simulink model "RocketTrajectory_TestModel"  (R2014a)
settings: Solver=ode3  StartTime=0.0  StopTime=25  FixedStep=0.01  MinStep=0.01  RelTol=1e-3
undefined symbols (not defined in the file or in its folder): area_rocket_planform, distance_tip_to_COP, dry_motor_weight, dry_rocket_cog, dry_rocket_weight, ground_launch_altitude, ground_pressure_ambient, ground_temperature_ambient, launch_angle, mass_flow_rate, moment_inertia_rocket, wet_motor_mass, wet_motor_weight
libraries: rocket_vertical_flight_library x4, rocket_drag_library x3, rocket_isa_model_library x2, rocket_dynamic_data_library x2, rocket_angular_flight_library x2
settings Model: Creator=scorpii  LastModifiedBy=scorpii
settings SolverCC: InitialStep=0.01
settings DataIOCC: LimitDataPoints=off
settings OptimizationCC: SimCompilerOptimization=off
settings DebuggingCC: ArtificialAlgebraicLoopMsg=error  MergeDetectMultiDrivingBlocksExec=error  FrameProcessingCompatibilityMsg=error
settings RTWCC: RTWCompilerOptimization=off

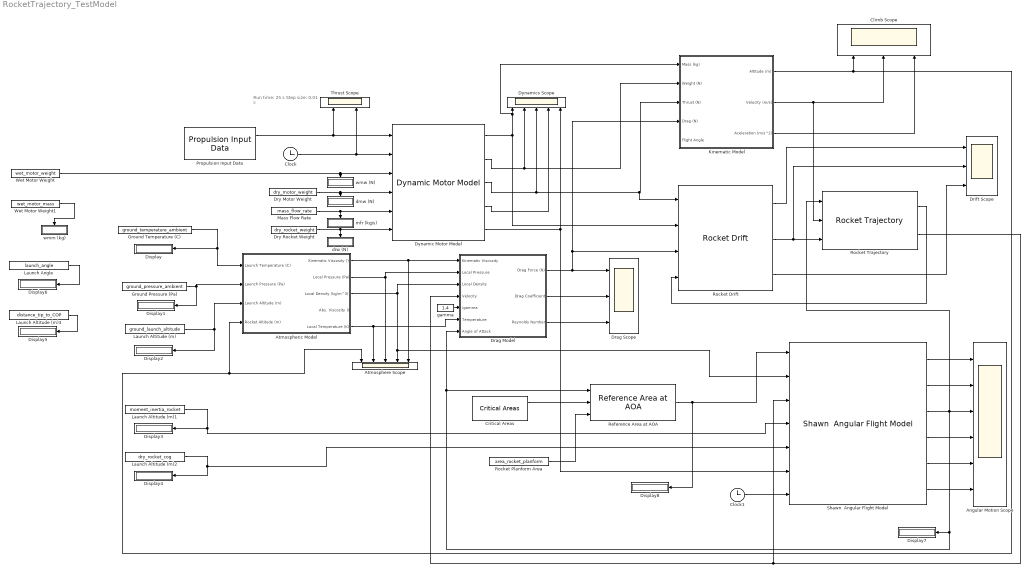
== system RocketTrajectory_TestModel ==
  note: Run time: 25 s
      | Step size: 0.01 s
  " Launch Angle" : Constant  Value=launch_angle
  Angular Motion Scope : Scope  NumInputPorts=6
      settings: TimeRange=10  YMin=-0.7~-0.125~-0.015~0.05~9~-5  YMax=0.9~0.125~0.015~0.275~24~5  SaveName=ScopeData5
  Atmosphere Scope : Scope  NumInputPorts=5
      settings: YMin=-1~28.5~96258.8~11.1784~-1.12485e-07  YMax=1~31.5~106391~12.355~-1.01773e-07  SaveName=ScopeData4
  Atmospheric Model : Subsystem
  Climb Scope : Scope  NumInputPorts=3
      settings: YMin=5.2~32.5~103.575  YMax=7~37.75~104.15
  Clock : Clock
  Clock1 : Clock
  Critical Areas : rocket_drag_library/Critical Areas
  Display{,1..8} (9 alike) : Display
  Drag Model : Subsystem
  Drag Scope : Scope  NumInputPorts=3
      settings: YMin=30~0.45~1.75e+07  YMax=240~0.725~5e+07  SaveName=ScopeData3
  Drift Scope : Scope  NumInputPorts=3
      settings: YMin=5.2~32.5~103.575  YMax=7~37.75~104.15  SaveName=ScopeData6
  Dry Motor Weight : Constant  Value=dry_motor_weight
  Dry Rocket Weight : Constant  Value=dry_rocket_weight
  Dynamic Motor Model : rocket_dynamic_data_library/Dynamic Motor Model
  Dynamics Scope : Scope  NumInputPorts=5
      settings: YMin=126.243~1238.44~774.486~-5~-5  YMax=139.531~1368.8~856.01~5~5
  Ground Pressure (Pa) : Constant  Value=ground_pressure_ambient
  Ground Temperature (C) : Constant  Value=ground_temperature_ambient
  Kinematic Model : Subsystem
  Launch Altitude (m) : Constant  Value=ground_launch_altitude
  Launch Altitude (m)1 : Constant  Value=moment_inertia_rocket
  Launch Altitude (m)2 : Constant  Value=dry_rocket_cog
  Launch Altitude (m)3 : Constant  Value=distance_tip_to_COP
  Mass Flow Rate : Constant  Value=mass_flow_rate
  Propulsion Input Data : rocket_dynamic_data_library/Propulsion Input Data
  Reference Area at AOA : rocket_angular_flight_library/Reference Area at AOA
  Rocket Drift : rocket_vertical_flight_library/Rocket Drift
  Rocket Planform Area : Constant  Value=area_rocket_planform
  Rocket Trajectory : rocket_vertical_flight_library/Rocket Trajectory
  Shawn  Angular Flight Model : rocket_angular_flight_library/Shawn  Angular Flight Model
  Thrust Scope : Scope  NumInputPorts=2
      settings: YMin=126.243~1238.44  YMax=139.531~1368.8  SaveName=ScopeData2
  "Wet Motor Weight " : Constant  Value=wet_motor_weight
  Wet Motor Weight1 : Constant  Value=wet_motor_mass
  dmw (N) : Display
  drw (N) : Display
  gamma : Constant  Value=1.4
  mfr (kg/s) : Display
  wmm (kg) : Display
  wmw (N) : Display
  wires:
  Drag Model/1(Drag Force (N)) -> Drag Scope/1, Rocket Drift/3, Kinematic Model/4(Drag (N))
  Clock/1 -> Dynamic Motor Model/2, Thrust Scope/2
  Kinematic Model/1(Altitude (m)) -> Climb Scope/1, Atmosphere Scope/1, Atmospheric Model/4(Rocket Altitude (m))
  Kinematic Model/2(Velocity (m/s)) -> Climb Scope/2, Rocket Trajectory/2
  Kinematic Model/3(Aceleration (m/s^2)) -> Climb Scope/3
  Atmospheric Model/3(Local Density (kg/m^3)) -> Shawn  Angular Flight Model/2, Atmosphere Scope/4, Drag Model/3(Local Density)
  Atmospheric Model/2(Local Pressure (Pa)) -> Atmosphere Scope/3, Drag Model/2(Local Pressure)
  Atmospheric Model/1(Kinematic Viscosity ()) -> Atmosphere Scope/5, Drag Model/1(Kinematic Viscosity)
  Atmospheric Model/5(Local Temperature (K)) -> Atmosphere Scope/2, Drag Model/6(Temperature)
  Dynamic Motor Model/2 -> Kinematic Model/2(Weight (N)), Dynamics Scope/2
  Dynamic Motor Model/1 -> Rocket Drift/2, Kinematic Model/1(Mass (kg)), Dynamics Scope/1
  Dynamic Motor Model/3 -> Rocket Drift/1, Kinematic Model/3(Thrust (N)), Dynamics Scope/3
  Propulsion Input Data/1 -> Dynamic Motor Model/1, Thrust Scope/1
  "Wet Motor Weight "/1 -> Dynamic Motor Model/3, wmw (N)/1
  Dry Motor Weight/1 -> Dynamic Motor Model/4, dmw (N)/1
  Mass Flow Rate/1 -> Dynamic Motor Model/5, mfr (kg/s)/1
  Drag Model/2(Drag Coefficient) -> Drag Scope/2
  Drag Model/3(Reynolds Number) -> Drag Scope/3
  gamma/1 -> Drag Model/5(\gamma)
  Ground Temperature (C)/1 -> Display/1, Atmospheric Model/1(Launch Temperature (C))
  Ground Pressure (Pa)/1 -> Display1/1, Atmospheric Model/2(Launch Pressure (Pa))
  Launch Altitude (m)/1 -> Atmospheric Model/3(Launch Altitude (m)), Display2/1
  Dynamic Motor Model/4 -> Dynamics Scope/4
  Dry Rocket Weight/1 -> Dynamic Motor Model/6, drw (N)/1
  Launch Altitude (m)1/1 -> Display3/1, Shawn  Angular Flight Model/4
  Shawn  Angular Flight Model/3 -> Rocket Trajectory/1, Display7/1, Drag Model/7(Angle of Attack), Reference Area at AOA/1, Angular Motion Scope/3
  Launch Altitude (m)2/1 -> Shawn  Angular Flight Model/5, Display4/1
  Launch Altitude (m)3/1 -> Display5/1
  Rocket Planform Area/1 -> Reference Area at AOA/3
  Critical Areas/1 -> Reference Area at AOA/2
  " Launch Angle"/1 -> Display6/1
  Shawn  Angular Flight Model/2 -> Angular Motion Scope/2
  Shawn  Angular Flight Model/1 -> Angular Motion Scope/1
  Wet Motor Weight1/1 -> wmm (kg)/1
  Reference Area at AOA/1 -> Display8/1, Shawn  Angular Flight Model/1
  Dynamic Motor Model/5 -> Shawn  Angular Flight Model/6, Dynamics Scope/5
  Clock1/1 -> Shawn  Angular Flight Model/7
  Shawn  Angular Flight Model/5 -> Angular Motion Scope/5
  Shawn  Angular Flight Model/4 -> Angular Motion Scope/4
  Shawn  Angular Flight Model/6 -> Angular Motion Scope/6
  Rocket Trajectory/1 -> Rocket Drift/4
  Rocket Drift/2 -> Drift Scope/2, Rocket Trajectory/3
  Rocket Trajectory/2 -> Shawn  Angular Flight Model/3, Drag Model/4(Velocity)
  Rocket Drift/1 -> Drift Scope/1
  Rocket Drift/3 -> Drift Scope/3

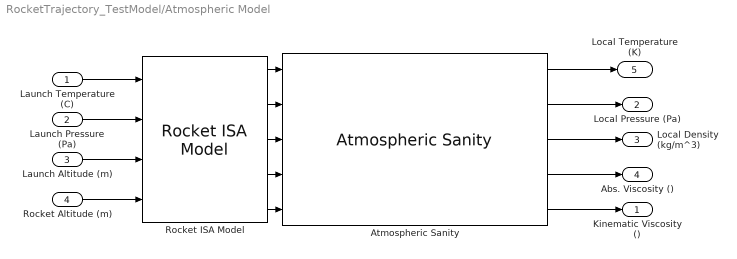
== system RocketTrajectory_TestModel/Atmospheric Model ==
  Launch Temperature (C) : Inport
  Launch Pressure (Pa) : Inport  Port=2
  Launch Altitude (m) : Inport  Port=3
  Rocket Altitude (m) : Inport  Port=4
  Atmospheric Sanity : rocket_isa_model_library/Atmospheric Sanity
  Rocket ISA Model : rocket_isa_model_library/Rocket ISA Model
  Kinematic Viscosity () : Outport
  Local Pressure (Pa) : Outport  Port=2
  Local Density (kg/m^3) : Outport  Port=3
  Abs. Viscosity () : Outport  Port=4
  Local Temperature (K) : Outport  Port=5
  wires:
  Rocket ISA Model/5 -> Atmospheric Sanity/5
  Rocket ISA Model/2 -> Atmospheric Sanity/2
  Rocket ISA Model/3 -> Atmospheric Sanity/3
  Atmospheric Sanity/2 -> Local Pressure (Pa)/1
  Rocket ISA Model/4 -> Atmospheric Sanity/4
  Atmospheric Sanity/5 -> Kinematic Viscosity ()/1
  Atmospheric Sanity/1 -> Local Temperature (K)/1
  Atmospheric Sanity/3 -> Local Density (kg/m^3)/1
  Rocket ISA Model/1 -> Atmospheric Sanity/1
  Launch Temperature (C)/1 -> Rocket ISA Model/1
  Atmospheric Sanity/4 -> Abs. Viscosity ()/1
  Launch Pressure (Pa)/1 -> Rocket ISA Model/2
  Launch Altitude (m)/1 -> Rocket ISA Model/3
  Rocket Altitude (m)/1 -> Rocket ISA Model/4

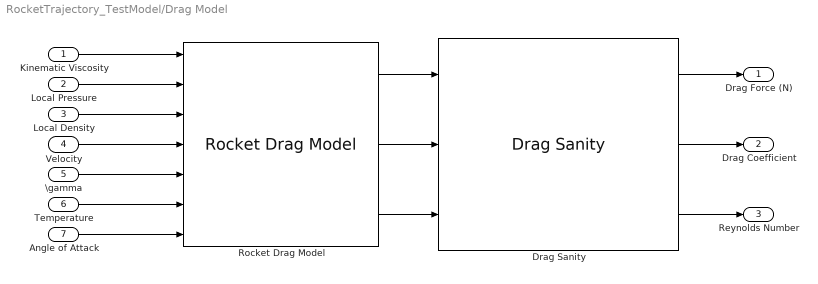
== system RocketTrajectory_TestModel/Drag Model ==
  Kinematic Viscosity : Inport
  Local Pressure : Inport  Port=2
  Local Density : Inport  Port=3
  Velocity : Inport  Port=4
  \gamma : Inport  Port=5
  Temperature : Inport  Port=6
  Angle of Attack : Inport  Port=7
  Drag Sanity : rocket_drag_library/Drag Sanity
  Rocket Drag Model : rocket_drag_library/Rocket Drag Model
      link override Drag Force/BasicDrag: MATLABFcn=BasicDrag
      link override Rocket Drag Coefficient/Skin Friction Drag Coefficient/area_fin_frontal: Value=area_fin_frontal
      link override Skin Friction Drag Coefficient/Actual Reynolds Number/Reynolds Number (Actual): MATLABFcn=ReynoldsNumberActual
  Drag Force (N) : Outport
  Drag Coefficient : Outport  Port=2
  Reynolds Number : Outport  Port=3
  wires:
  Local Pressure/1 -> Rocket Drag Model/2
  Kinematic Viscosity/1 -> Rocket Drag Model/1
  Local Density/1 -> Rocket Drag Model/3
  Rocket Drag Model/3 -> Drag Sanity/3
  Rocket Drag Model/2 -> Drag Sanity/2
  Rocket Drag Model/1 -> Drag Sanity/1
  Drag Sanity/1 -> Drag Force (N)/1
  Drag Sanity/2 -> Drag Coefficient/1
  Drag Sanity/3 -> Reynolds Number/1
  Temperature/1 -> Rocket Drag Model/6
  Velocity/1 -> Rocket Drag Model/4
  \gamma/1 -> Rocket Drag Model/5
  Angle of Attack/1 -> Rocket Drag Model/7

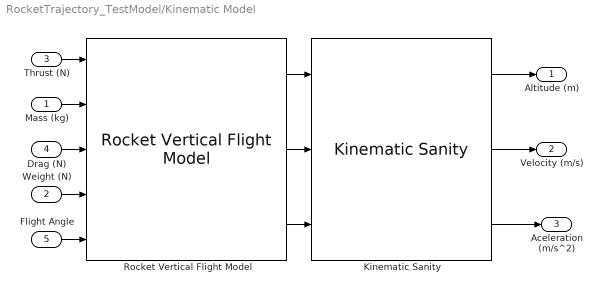
== system RocketTrajectory_TestModel/Kinematic Model ==
  Mass (kg) : Inport
  Weight (N) : Inport  Port=2
  Thrust (N) : Inport  Port=3
  Drag (N) : Inport  Port=4
  Flight Angle : Inport  Port=5
  Kinematic Sanity : rocket_vertical_flight_library/Kinematic Sanity
  Rocket Vertical Flight Model : rocket_vertical_flight_library/Rocket Vertical Flight Model
  Altitude (m) : Outport
  Velocity (m/s) : Outport  Port=2
  Aceleration (m/s^2) : Outport  Port=3
  wires:
  Rocket Vertical Flight Model/2 -> Kinematic Sanity/2
  Kinematic Sanity/2 -> Velocity (m/s)/1
  Rocket Vertical Flight Model/1 -> Kinematic Sanity/1
  Kinematic Sanity/3 -> Aceleration (m/s^2)/1
  Kinematic Sanity/1 -> Altitude (m)/1
  Rocket Vertical Flight Model/3 -> Kinematic Sanity/3
  Mass (kg)/1 -> Rocket Vertical Flight Model/2
  Weight (N)/1 -> Rocket Vertical Flight Model/4
  Thrust (N)/1 -> Rocket Vertical Flight Model/1
  Drag (N)/1 -> Rocket Vertical Flight Model/3
  Flight Angle/1 -> Rocket Vertical Flight Model/5
